simulink model "SwitchedReluctanceMotor"  (R2014a)
settings: Solver=FixedStepDiscrete  StartTime=0.0  StopTime=0.35  FixedStep=Ts  RelTol=1e-3  AbsTol=1e-5
PreLoadFcn:
  | Ts=1e-6;
  | load srm64_60kw
undefined symbols (not defined in the file): DiscIntNeverNeededParam, find_system
libraries: powerlib x15
Description:
  | Copyright 2008-2014 The MathWorks, Inc.
settings Model: ExtModeAutoUpdateStatusClock=off  Creator=MathWorks  LastModifiedBy=usmankhan
settings SolverCC: InsertRTBMode=Auto
settings DataIOCC: SignalLoggingSaveFormat=ModelDataLogs  SignalLoggingName=sigsOut
settings OptimizationCC: ExpressionDepthLimit=2147483647  InitFltsAndDblsToZero=on
settings DebuggingCC: UnderspecifiedInitializationDetection=Classic  CheckExecutionContextPreStartOutputMsg=on  CheckExecutionContextRuntimeOutputMsg=on  SignalResolutionControl=TryResolveAllWithWarning  SolverPrmCheckMsg=none  MultiTaskDSMMsg=warning  MultiTaskCondExecSysMsg=none  FcnCallInpInsideContextMsg=UseLocalSettings  StateNameClashWarn=warning
settings HardwareCC: TargetUnknown=on
settings RTWCC: IncludeERTFirstTime=on
settings GRTTargetCC: CombineOutputUpdateFcns=off  GRTInterface=on

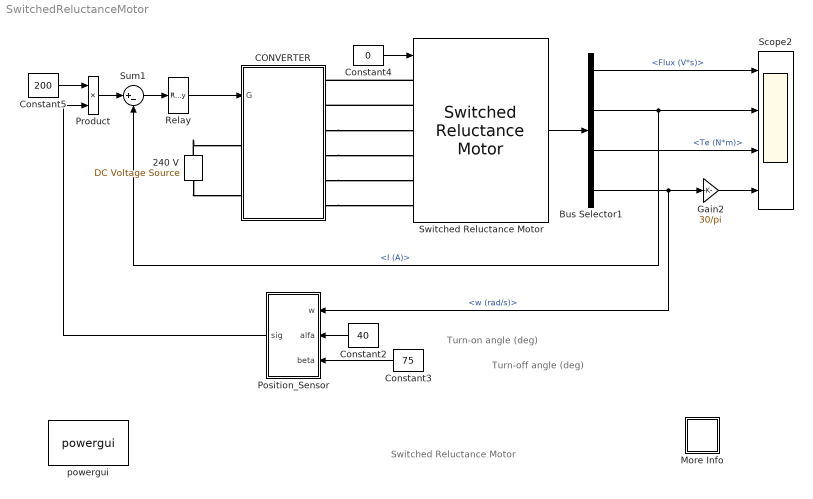
== system SwitchedReluctanceMotor ==
  note: Turn-off angle (deg)
  note: Turn-on angle (deg)
  note: Switched Reluctance Motor
  240 V : powerlib/Electrical Sources/DC Voltage Source  Amplitude=240  Measurements=None
  Bus Selector1 : BusSelector  OutputSignals=Flux (V*s),I (A),Te (N*m),w (rad/s)
  CONVERTER : Subsystem  LoadFcn=find_system(gcs,'FollowLinks', 'on', 'LookUnderMasks', 'all');
  Constant2 : Constant  Value=40
  Constant3 : Constant  Value=75
  Constant4 : Constant  Value=0
  Constant5 : Constant  Value=200
  Gain2 : Gain  Gain=30/pi  SaturateOnIntegerOverflow=on  OutDataTypeStr=Inherit: Same as input  ParamDataTypeStr=Inherit: Same as input
  More Info : Subsystem
      settings: OpenFcn=showdemo(bdroot(gcb))
      mask Display: disp('?')
  Position_Sensor : Subsystem
  Product : Product  SaturateOnIntegerOverflow=on  OutDataTypeStr=Inherit: Same as first input
  Relay : Relay  OnSwitchValue=10  OffSwitchValue=-10  SampleTime=Ts
  Scope2 : Scope  NumInputPorts=4
      settings: TimeRange=0.35  YMin=-0.2~-100~0~0  YMax=0.6000000000000001~300~150~5000  SaveName=VI  Decimation=10
  Sum1 : Sum  Inputs=|+-  SaturateOnIntegerOverflow=on
  Switched Reluctance Motor : powerlib/Machines/Switched Reluctance Motor  MachineType=6/4  MachineModel=Specific model  StatorResistance=0.05  PlotCurves=off  Inertia=0.05  Friction=0.02  InitialSpeed=[0,0]  Lq=0.67e-3  Ld=23.6e-3  Lsat=0.15e-3  MaximumCurrent=450  MaximumFluxLinkage=0.486  MagnetisationCharacteristic='srm64_60kw.mat'  RotorAngleVector=[0 10 20 30 40 45]  StatorCurrentVector=0:25:450  TsPowergui=0  TsBlock=-1
  powergui : powerlib/powergui  Priority=2  SimulationMode=Discrete  SolverType=Tustin  SampleTime=Ts  frequency=60  SPID=off  DisableSnubberDevices=off  DisableRonSwitches=off  DisableVfSwitches=off  SwTol=0  Interpol=off  DisplayEquations=off  Ts=0  methode=off  frequencyindice=0  Pbase=100e6  ErrMax=1e-4  Iterations=50  UnitsV=kV  UnitsW=MW  FunctionMessages=off  echomessages=off  HookPort=off  EnableUseOfTLC=off  x0status=blocks  RestoreLinks=warning  ResistiveCurrentMeasurement=off  Frange=[0:2:500]  Ylog=off  Xlog=on  ShowGrid=off  save=off  variable=ZData  structure=0  ZoomFFT=on  StartTime=0.0  cycles=1  DisplayStyle=1  fundamental=60  FreqAxis=off  MaxFrequency=1000  frequencyindicesteady=1  RmsSteady=1  display=off
  wires:
  Constant2/1 -> Position_Sensor/2(alfa)
  Constant3/1 -> Position_Sensor/3(beta)
  Constant4/1 -> Switched Reluctance Motor/1
  Sum1/1 -> Relay/1
  Product/1 -> Sum1/1
  Constant5/1 -> Product/1
  Position_Sensor/1(sig) -> Product/2
  Relay/1 -> CONVERTER/1(G)
  Switched Reluctance Motor/1 -> Bus Selector1/1
  Bus Selector1/1 -> Scope2/1  "<Flux (V*s)>"
  Bus Selector1/2 -> Scope2/2, Sum1/2  "<I (A)>"
  Bus Selector1/3 -> Scope2/3  "<Te (N*m)>"
  Gain2/1 -> Scope2/4
  Bus Selector1/4 -> Gain2/1, Position_Sensor/1(w)  "<w (rad/s)>"
  connections:
  240 V/RConn1 -- CONVERTER/LConn1
  240 V/LConn1 -- CONVERTER/LConn2
  Switched Reluctance Motor/LConn1 -- CONVERTER/RConn1
  Switched Reluctance Motor/LConn2 -- CONVERTER/RConn2
  CONVERTER/RConn3 -- Switched Reluctance Motor/LConn3
  CONVERTER/RConn4 -- Switched Reluctance Motor/LConn4
  CONVERTER/RConn5 -- Switched Reluctance Motor/LConn5
  CONVERTER/RConn6 -- Switched Reluctance Motor/LConn6

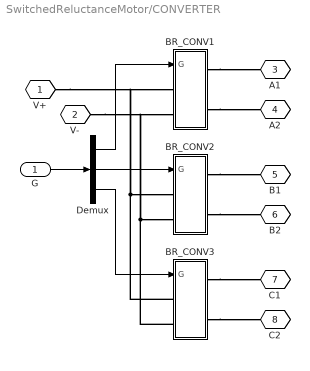
== system SwitchedReluctanceMotor/CONVERTER ==
  G : Inport
  BR_CONV1 : Subsystem
  BR_CONV2 : Subsystem
  BR_CONV3 : Subsystem
  Demux : Demux  Outputs=3
  V+ : PMIOPort  Tag=PMCPort  Port=1  Side=Left
  V- : PMIOPort  Tag=PMCPort  Port=2  Side=Left
  A1 : PMIOPort  Tag=PMCPort  Port=3  Side=Right
  A2 : PMIOPort  Tag=PMCPort  Port=4  Side=Right
  B1 : PMIOPort  Tag=PMCPort  Port=5  Side=Right
  B2 : PMIOPort  Tag=PMCPort  Port=6  Side=Right
  C1 : PMIOPort  Tag=PMCPort  Port=7  Side=Right
  C2 : PMIOPort  Tag=PMCPort  Port=8  Side=Right
  wires:
  Demux/3 -> BR_CONV3/1(G)
  Demux/1 -> BR_CONV1/1(G)
  Demux/2 -> BR_CONV2/1(G)
  G/1 -> Demux/1
  connections:
  BR_CONV3/RConn2 -- C2/RConn1
  BR_CONV3/RConn1 -- C1/RConn1
  BR_CONV2/RConn2 -- B2/RConn1
  BR_CONV2/RConn1 -- B1/RConn1
  BR_CONV1/RConn2 -- A2/RConn1
  BR_CONV1/RConn1 -- A1/RConn1
  BR_CONV3/LConn2 -- BR_CONV1/LConn2 -- V-/RConn1 -- BR_CONV2/LConn2
  BR_CONV3/LConn1 -- BR_CONV1/LConn1 -- V+/RConn1 -- BR_CONV2/LConn1

== system SwitchedReluctanceMotor/More Info ==

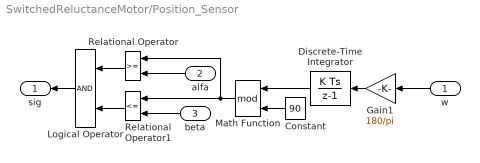
== system SwitchedReluctanceMotor/Position_Sensor ==
  w : Inport
  alfa : Inport  Port=2
  beta : Inport  Port=3
  Constant : Constant  Value=90
  Discrete-Time Integrator : DiscreteIntegrator  InitialCondition=[0 -30 -60]  SampleTime=Ts  ICPrevOutput=DiscIntNeverNeededParam  ICPrevScaledInput=DiscIntNeverNeededParam
  Gain1 : Gain  Gain=180/pi  SaturateOnIntegerOverflow=on  OutDataTypeStr=Inherit: Same as input  ParamDataTypeStr=Inherit: Same as input
  Logical Operator : Logic  AllPortsSameDT=off
  Math Function : Math  Operator=mod  SaturateOnIntegerOverflow=on
  Relational Operator : RelationalOperator
  Relational Operator1 : RelationalOperator  Operator=<=
  sig : Outport
  wires:
  Logical Operator/1 -> sig/1
  w/1 -> Gain1/1
  Math Function/1 -> Relational Operator/1, Relational Operator1/1
  Relational Operator1/1 -> Logical Operator/2
  Gain1/1 -> Discrete-Time Integrator/1
  beta/1 -> Relational Operator1/2
  alfa/1 -> Relational Operator/2
  Relational Operator/1 -> Logical Operator/1
  Constant/1 -> Math Function/2
  Discrete-Time Integrator/1 -> Math Function/1

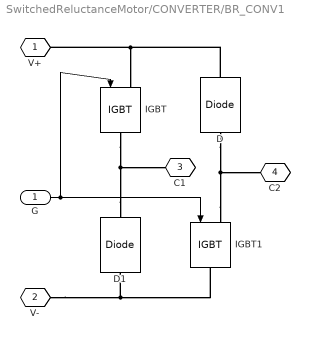
== system SwitchedReluctanceMotor/CONVERTER/BR_CONV1 ==
  G : Inport
  D : powerlib/Power Electronics/Diode  Ron=1e-3  Lon=0  Vf=0.8  IC=0  UseSnubber=off  Rs=1000  Cs=inf  Measurements=off
  D1 : powerlib/Power Electronics/Diode  Ron=1e-3  Lon=0  Vf=0.8  IC=0  UseSnubber=off  Rs=1000  Cs=inf  Measurements=off
  IGBT : powerlib/Power Electronics/IGBT  Ron=1e-3  Lon=0  Vf=1  Tf=0  Tt=0  IC=0  Rs=200  Cs=0.1e-6  Measurements=off
  IGBT1 : powerlib/Power Electronics/IGBT  Ron=1e-3  Lon=0  Vf=1  Tf=0  Tt=0  IC=0  Rs=200  Cs=0.1e-6  Measurements=off
  V+ : PMIOPort  Tag=PMCPort  Port=1  Side=Left
  V- : PMIOPort  Tag=PMCPort  Port=2  Side=Left
  C1 : PMIOPort  Tag=PMCPort  Port=3  Side=Right
  C2 : PMIOPort  Tag=PMCPort  Port=4  Side=Right
  wires:
  G/1 -> IGBT/1, IGBT1/1
  connections:
  D1/LConn1 -- V-/RConn1 -- IGBT1/RConn1
  IGBT1/LConn1 -- D/LConn1 -- C2/RConn1
  D1/RConn1 -- IGBT/RConn1 -- C1/RConn1
  D/RConn1 -- V+/RConn1 -- IGBT/LConn1

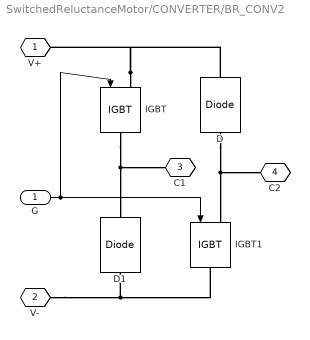
== system SwitchedReluctanceMotor/CONVERTER/BR_CONV2 ==
  G : Inport
  D : powerlib/Power Electronics/Diode  Ron=1e-3  Lon=0  Vf=0.8  IC=0  UseSnubber=off  Rs=1000  Cs=inf  Measurements=off
  D1 : powerlib/Power Electronics/Diode  Ron=1e-3  Lon=0  Vf=0.8  IC=0  UseSnubber=off  Rs=1000  Cs=inf  Measurements=off
  IGBT : powerlib/Power Electronics/IGBT  Ron=1e-3  Lon=0  Vf=1  Tf=0  Tt=0  IC=0  Rs=200  Cs=0.1e-6  Measurements=off
  IGBT1 : powerlib/Power Electronics/IGBT  Ron=1e-3  Lon=0  Vf=1  Tf=0  Tt=0  IC=0  Rs=200  Cs=0.1e-6  Measurements=off
  V+ : PMIOPort  Tag=PMCPort  Port=1  Side=Left
  V- : PMIOPort  Tag=PMCPort  Port=2  Side=Left
  C1 : PMIOPort  Tag=PMCPort  Port=3  Side=Right
  C2 : PMIOPort  Tag=PMCPort  Port=4  Side=Right
  wires:
  G/1 -> IGBT1/1, IGBT/1
  connections:
  IGBT/LConn1 -- V+/RConn1 -- D/RConn1
  IGBT/RConn1 -- D1/RConn1 -- C1/RConn1
  D/LConn1 -- IGBT1/LConn1 -- C2/RConn1
  V-/RConn1 -- D1/LConn1 -- IGBT1/RConn1

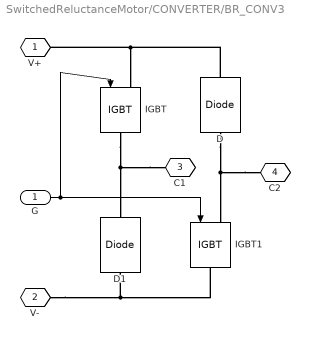
== system SwitchedReluctanceMotor/CONVERTER/BR_CONV3 ==
  G : Inport
  D : powerlib/Power Electronics/Diode  Ron=1e-3  Lon=0  Vf=0.8  IC=0  UseSnubber=off  Rs=1000  Cs=inf  Measurements=off
  D1 : powerlib/Power Electronics/Diode  Ron=1e-3  Lon=0  Vf=0.8  IC=0  UseSnubber=off  Rs=1000  Cs=inf  Measurements=off
  IGBT : powerlib/Power Electronics/IGBT  Ron=1e-3  Lon=0  Vf=1  Tf=0  Tt=0  IC=0  Rs=200  Cs=0.1e-6  Measurements=off
  IGBT1 : powerlib/Power Electronics/IGBT  Ron=1e-3  Lon=0  Vf=1  Tf=0  Tt=0  IC=0  Rs=200  Cs=0.1e-6  Measurements=off
  V+ : PMIOPort  Tag=PMCPort  Port=1  Side=Left
  V- : PMIOPort  Tag=PMCPort  Port=2  Side=Left
  C1 : PMIOPort  Tag=PMCPort  Port=3  Side=Right
  C2 : PMIOPort  Tag=PMCPort  Port=4  Side=Right
  wires:
  G/1 -> IGBT/1, IGBT1/1
  connections:
  IGBT1/RConn1 -- D1/LConn1 -- V-/RConn1
  C2/RConn1 -- IGBT1/LConn1 -- D/LConn1
  C1/RConn1 -- D1/RConn1 -- IGBT/RConn1
  D/RConn1 -- V+/RConn1 -- IGBT/LConn1
